simulink model "Seeker_detect"  (R2025b)
settings: Solver=FixedStepAuto  StartTime=0.0  StopTime=10.0  RelTol=1e-3
undefined symbols (not defined in the file): d_raycount, s_aperture_diameter, s_efficiency, s_fov, sal_atmos_coef
settings Model: DataDictionary=Seeker_detect_data.sldd  Creator=mauro  LastModifiedBy=mauro

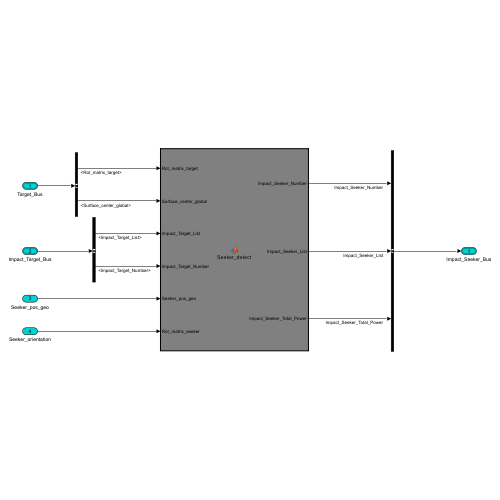
[thumbnail: Simulink's stored preview of the top-level diagram]
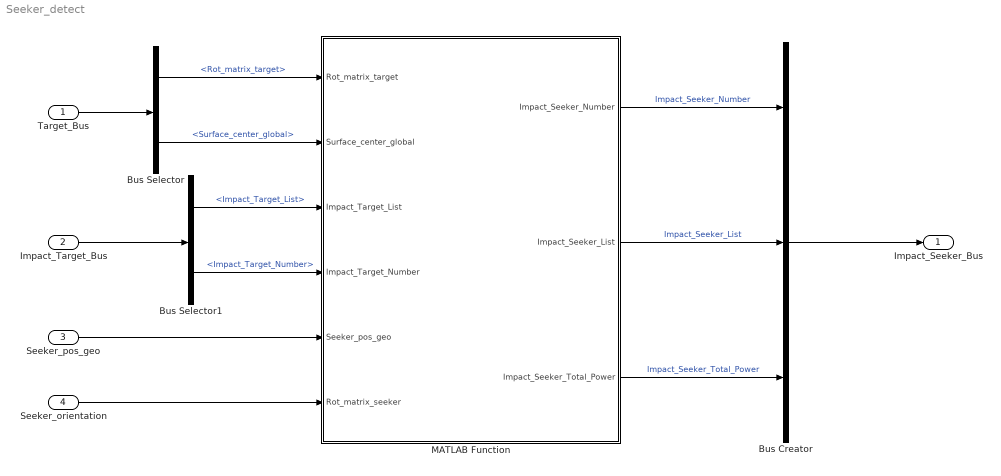
== system Seeker_detect ==
  Target_Bus : Inport  OutDataTypeStr=Bus: Target_bus
  Impact_Target_Bus : Inport  Port=2  OutDataTypeStr=Bus: Impact_Target_Bus
  Seeker_pos_geo : Inport  Port=3  PortDimensions=[3 1]
  Seeker_orientation : Inport  Port=4  PortDimensions=[3 3]
  Bus Creator : BusCreator  Inputs=3  OutDataTypeStr=Bus: Impact_Seeker_Bus  NonVirtualBus=on
  Bus Selector : BusSelector  OutputSignals=Rot_matrix_target,Surface_center_global
  Bus Selector1 : BusSelector  OutputSignals=Impact_Target_List,Impact_Target_Number
  MATLAB Function : MATLAB Function  TreatAsAtomicUnit=on
  Impact_Seeker_Bus : Outport  OutDataTypeStr=Bus: Impact_Seeker_Bus  BusOutputAsStruct=on
  wires:
  Seeker_pos_geo/1 -> MATLAB Function/5(Seeker_pos_geo)
  Target_Bus/1 -> Bus Selector/1
  Bus Selector/1 -> MATLAB Function/1(Rot_matrix_target)  "<Rot_matrix_target>"
  Bus Selector/2 -> MATLAB Function/2(Surface_center_global)  "<Surface_center_global>"
  Impact_Target_Bus/1 -> Bus Selector1/1
  Bus Selector1/1 -> MATLAB Function/3(Impact_Target_List)  "<Impact_Target_List>"
  Bus Selector1/2 -> MATLAB Function/4(Impact_Target_Number)  "<Impact_Target_Number>"
  MATLAB Function/3(Impact_Seeker_Total_Power) -> Bus Creator/3  "Impact_Seeker_Total_Power"
  MATLAB Function/2(Impact_Seeker_List) -> Bus Creator/2  "Impact_Seeker_List"
  MATLAB Function/1(Impact_Seeker_Number) -> Bus Creator/1  "Impact_Seeker_Number"
  Bus Creator/1 -> Impact_Seeker_Bus/1
  Seeker_orientation/1 -> MATLAB Function/6(Rot_matrix_seeker)

== matlab function Seeker_detect/MATLAB Function ==
  data: Rot_matrix_target input; Impact_Seeker_Number output; Surface_center_global input; Impact_Seeker_List output; Impact_Target_List input; Impact_Target_Number input; Seeker_pos_geo input; Impact_Seeker_Total_Power output; d_raycount parameter; sal_atmos_coef parameter; s_fov parameter; s_aperture_diameter parameter; s_efficiency parameter; Rot_matrix_seeker input
function [Impact_Seeker_Number,Impact_Seeker_List,Impact_Seeker_Total_Power]  = Seeker_detect(Rot_matrix_target,Surface_center_global,Impact_Target_List,Impact_Target_Number,Seeker_pos_geo,d_raycount, sal_atmos_coef,s_fov, s_aperture_diameter, s_efficiency, Rot_matrix_seeker)

    Impact_Seeker_Number = 0;% Total number of rays detected by the seeker for each laser pulse.
    Impact_Seeker_List = zeros(5,d_raycount);

    
    for i = 1:Impact_Target_Number
    
        if Impact_Target_List(4,i)==1
    
            Impact_Target_Point = Surface_center_global(:,1)+Rot_matrix_target*[0;Impact_Target_List(2,i);Impact_Target_List(3,i)];
            n_vector            = [-1;0;0];
    
        elseif Impact_Target_List(4,i)==2
    
            Impact_Target_Point = Surface_center_global(:,2)+Rot_matrix_target*[0;-Impact_Target_List(2,i);Impact_Target_List(3,i)];
            n_vector            = [1;0;0];
    
        elseif Impact_Target_List(4,i)==3
    
            Impact_Target_Point = Surface_center_global(:,3)+Rot_matrix_target*[-Impact_Target_List(2,i);0;Impact_Target_List(3,i)];
            n_vector            = [0;-1;0];
    
        elseif Impact_Target_List(4,i)==4
    
            Impact_Target_Point = Surface_center_global(:,4)+Rot_matrix_target*[Impact_Target_List(2,i);0;Impact_Target_List(3,i)];
            n_vector            = [0;1;0];
    
        elseif Impact_Target_List(4,i)==5
    
            Impact_Target_Point = Surface_center_global(:,5)+Rot_matrix_target*[-Impact_Target_List(3,i);Impact_Target_List(2,i);0];
            n_vector            = [0;0;-1];
    
        else
    
            Impact_Target_Point = Surface_center_global(:,5)+Rot_matrix_target*[-Impact_Target_List(3,i);-Impact_Target_List(2,i);0];
            n_vector            = [0;0;1];
    
        end
    
        st_vector           = Impact_Target_Point-Seeker_pos_geo;
        s_vector            = Rot_matrix_seeker*[1;0;0];
        n_vector_global     = Rot_matrix_target*n_vector;
        mu                  = acos(dot(s_vector,st_vector)/norm(s_vector)/norm(st_vector));
        alpha               = acos(dot(n_vector_global,-st_vector)/norm(n_vector_global)/norm(st_vector));
    
        if mu<=s_fov && alpha<=pi/2
    
            Impact_Seeker_Number  = Impact_Seeker_Number+1;
            st_vector_local       = Rot_matrix_seeker'*st_vector;
            Impact_Seeker_List(1,Impact_Seeker_Number) = norm(st_vector_local);
            Impact_Seeker_List(2,Impact_Seeker_Number) = -st_vector_local(2)/norm(st_vector_local);
            Impact_Seeker_List(3,Impact_Seeker_Number) = -st_vector_local(3)/norm(st_vector_local);
    
            u = Impact_Seeker_List(2,Impact_Seeker_Number);
            v = Impact_Seeker_List(3,Impact_Seeker_Number);   
    
            if u>=0 && v>=0
    
                Impact_Seeker_List(4,Impact_Seeker_Number) = 1; 
    
            elseif u>=0 && v<=0
    
                Impact_Seeker_List(4,Impact_Seeker_Number) = 2;
                
            elseif u<=0 && v<=0
    
                Impact_Seeker_List(4,Impact_Seeker_Number) = 3;
    
            elseif u<=0 && v>=0
    
                Impact_Seeker_List(4,Impact_Seeker_Number) = 4;
    
            end
    
            Radiant_Intensity_Seeker                    = Impact_Target_List(5,i)*cos(alpha)/pi;
            Impact_Seeker_List(5,Impact_Seeker_Number)  = Radiant_Intensity_Seeker*pi*(s_aperture_diameter/2)^2/Impact_Seeker_List(1,Impact_Seeker_Number)^2*cos(mu)*s_efficiency*exp(-sal_atmos_coef*Impact_Seeker_List(1,Impact_Seeker_Number));
       
        end
    
    end
    
    Impact_Seeker_Total_Power   = sum(Impact_Seeker_List(5,:));

end
